simulink model "InterpolationQerr"  (R2019b)
settings: Solver=VariableStepDiscrete  StartTime=0.0  StopTime=16  MaxStep=0.01  RelTol=1e-3
values from neighbouring files (symbols this model uses):
  sim_Acc = Acc(jj)    [findDiscreteIntegrationError.m]
  sim_endQ = endQ(ii)    [findDiscreteIntegrationError.m]
  sim_endTime = 15    [findDiscreteIntegrationError.m]
  sim_startQ = 0    [findDiscreteIntegrationError.m]
  sim_startTime = 0    [findDiscreteIntegrationError.m]
undefined symbols (not defined in the file or in its folder): DiscIntNeverNeededParam
settings Model: Creator=Aljaz  LastModifiedBy=Aljaz
settings DataIOCC: SaveOutput=off  SaveTime=off  ReturnWorkspaceOutputs=off

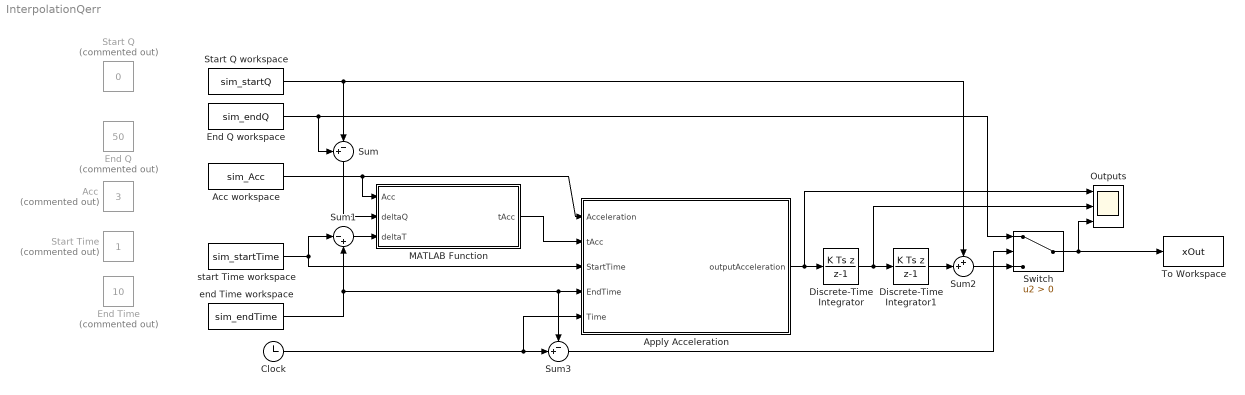
== system InterpolationQerr ==
  Acc : Constant  Commented=on  Value=3
  Acc workspace : Constant  Value=sim_Acc
  Apply Acceleration : Subsystem
  Clock : Clock
  Discrete-Time Integrator : DiscreteIntegrator  IntegratorMethod=Integration: Backward Euler  SampleTime=-1  ICPrevOutput=DiscIntNeverNeededParam  ICPrevScaledInput=DiscIntNeverNeededParam
  Discrete-Time Integrator1 : DiscreteIntegrator  IntegratorMethod=Integration: Backward Euler  SampleTime=-1  ICPrevOutput=DiscIntNeverNeededParam  ICPrevScaledInput=DiscIntNeverNeededParam
  End Q : Constant  Commented=on  Value=50
  End Q workspace : Constant  Value=sim_endQ
  End Time : Constant  Commented=on  Value=10
  MATLAB Function : MATLAB Function  TreatAsAtomicUnit=on
  Outputs : Scope  NumInputPorts=3
  Start Q : Constant  Commented=on  Value=0
  Start Q workspace : Constant  Value=sim_startQ
  Start Time : Constant  Commented=on
  Sum : Sum  Inputs=+-|
  Sum1 : Sum  Inputs=|-+
  Sum2 : Sum  Inputs=++|
  Sum3 : Sum  Inputs=-+|
  Switch : Switch  Criteria=u2 > Threshold
  To Workspace : ToWorkspace  VariableName=xOut  SampleTime=-1
  end Time workspace : Constant  Value=sim_endTime
  start Time workspace : Constant  Value=sim_startTime
  wires:
  Acc workspace/1 -> MATLAB Function/1(Acc), Apply Acceleration/1(Acceleration)
  start Time workspace/1 -> Apply Acceleration/3(StartTime), Sum1/1
  end Time workspace/1 -> Sum3/1, Apply Acceleration/4(EndTime), Sum1/2
  Clock/1 -> Sum3/2, Apply Acceleration/5(Time)
  Apply Acceleration/1(outputAcceleration) -> Outputs/1, Discrete-Time Integrator/1
  Discrete-Time Integrator/1 -> Outputs/2, Discrete-Time Integrator1/1
  Sum/1 -> MATLAB Function/2(deltaQ)
  Sum1/1 -> MATLAB Function/3(deltaT)
  MATLAB Function/1(tAcc) -> Apply Acceleration/2(tAcc)
  Start Q workspace/1 -> Sum/2, Sum2/1
  End Q workspace/1 -> Sum/1, Switch/1
  Discrete-Time Integrator1/1 -> Sum2/2
  Sum2/1 -> Switch/3
  Sum3/1 -> Switch/2
  Switch/1 -> To Workspace/1, Outputs/3

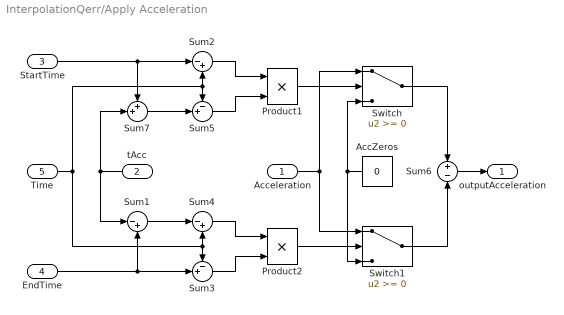
== system InterpolationQerr/Apply Acceleration ==
  Acceleration : Inport
  tAcc : Inport  Port=2
  StartTime : Inport  Port=3
  EndTime : Inport  Port=4
  Time : Inport  Port=5
  AccZeros : Constant  Value=0
  Product1 : Product
  Product2 : Product
  Sum1 : Sum  Inputs=|-+
  Sum2 : Sum  Inputs=|-+
  Sum3 : Sum  Inputs=-+|
  Sum4 : Sum  Inputs=|-+
  Sum5 : Sum  Inputs=-+|
  Sum6 : Sum  Inputs=+|-
  Sum7 : Sum  Inputs=++|
  Switch : Switch
  Switch1 : Switch
  outputAcceleration : Outport
  wires:
  Switch/1 -> Sum6/1
  Acceleration/1 -> Switch/1, Switch1/1
  Switch1/1 -> Sum6/2
  Product1/1 -> Switch/2
  AccZeros/1 -> Switch/3, Switch1/3
  Sum6/1 -> outputAcceleration/1
  Sum2/1 -> Product1/1
  Sum5/1 -> Product1/2
  Time/1 -> Sum4/2, Sum3/1, Sum2/2, Sum5/1
  StartTime/1 -> Sum7/1, Sum2/1
  tAcc/1 -> Sum1/1, Sum7/2
  Sum7/1 -> Sum5/2
  EndTime/1 -> Sum1/2, Sum3/2
  Sum1/1 -> Sum4/1
  Sum4/1 -> Product2/1
  Sum3/1 -> Product2/2
  Product2/1 -> Switch1/2

== matlab function InterpolationQerr/MATLAB Function ==
  data: Acc input; deltaQ input; tAcc output; deltaT input
function tAcc = getAccTime(Acc,deltaQ,deltaT)

D=deltaT.^2.*Acc-4*deltaQ;
D=D./Acc;
tAcc=deltaT/2-0.5*sqrt(D);
end
